simulink model "codificacion_y_modulacion_new"  (R2024b)
settings: Solver=VariableStepAuto  StartTime=0.0  StopTime=inf  RelTol=1e-3
undefined symbols (not defined in the file or in its folder): r
settings Model: SnapshotBufferSize=1000  SnapshotInterval=1000  Creator=SALA 321  LastModifiedBy=SALA 321

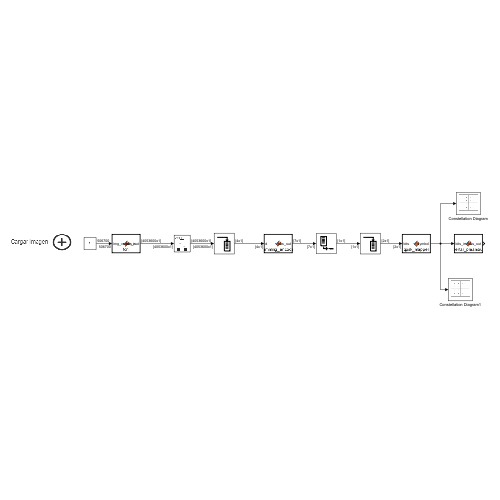
[thumbnail: Simulink's stored preview of the top-level diagram]
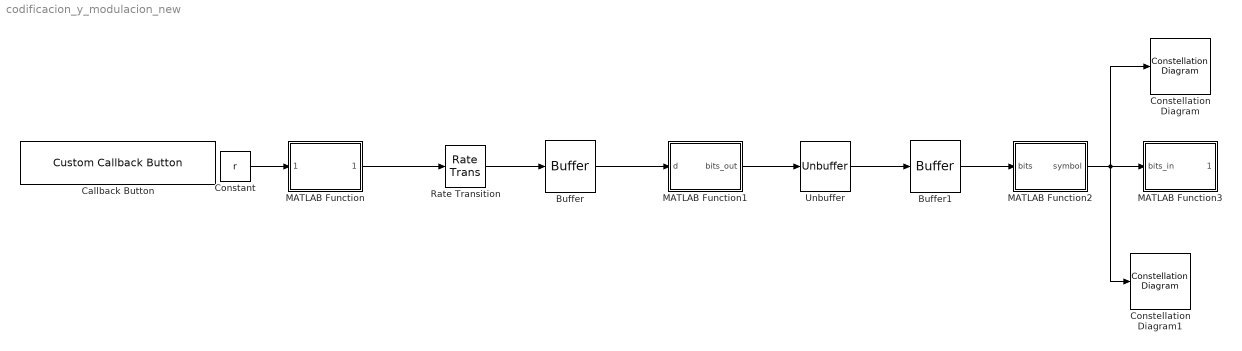
== system codificacion_y_modulacion_new ==
  Buffer : Buffer  N=4  OutputFrames=off
  Buffer1 : Buffer  N=2  OutputFrames=off
  Callback Button : CustomCallbackButton  Configuration="{\"components\":[{\"name\":\"BackgroundImageComponent\",\"settings\":{\"image\":{\"size\":[0,0],\"src\":\"default\",\"srcOrientation\":\"horizontal\"},\"position\":[0,0,1,1],\"scaleMode\":\"0\"}},{\"name\":\"ButtonStateComponent\",\"settings\":{\"buttonType\":\"momentary\",\"clickFcn\":\"[archivo, ruta] = uigetfile( ...\\n    {'*.jpg;*.jpeg;*.png;*.bmp;*.tif;*.tiff;*.gif;*.webp;*.jfif', ...\\n     'Archivos de imagen'}, ...\\n     'Seleccionar imagen');\\n\\nif isequal(archivo,0)\\n    disp('No se seleccionó imagen');\\n    return;\\nend\\n\\nrutaCompleta = fullfile(ruta, archivo);\\n\\ntry\\n    img = imread(rutaCompleta);\\ncatch\\n    errordlg('Formato no soportado por la versión de MATLAB','Error');\\n    return;\\nend\\n\\nif ndims(img) ~= 3 || size(img,3) ~= 3\\n    errordlg('La imagen debe ser RGB','Error');\\n    return;\\nend\\n\\n\\nalto = size(img,1);\\nancho = size(img,2);\\n\\nif alto < 492 || ancho < 740\\n    errordlg('La imagen debe tener mínimo 740x492 pixeles','Error');\\n    return;\\nend\\n\\nimgGray = rgb2gray(img);\\n\\nniveles = 16;              % Número de niveles de cuantización\\ndelta = 256\\/niveles;       % Paso de cuantización\\n\\nimgCuant = floor(double(img)\\/delta)*delta + delta\\/2;\\nimgCuant = uint8(imgCuant);\\n\\nassignin('base','imagen_original',img);\\nassignin('base','imagen_gris',imgGray);\\nassignin('base','imagen_cuantizada',imgCuant);\\n\\nr = reshape(imgGray,1,[]);\\nassignin('base','r',r);\\n\\ndisp(['Imagen cargada correctamente: ', archivo]);\\ndisp(['Tamaño: ', num2str(ancho), 'x', num2str(alto)]);\\ndisp(['Vector serializado r → tamaño: ', mat2str(size(r))]);\\n\\nfigure(2)\\nsubplot(1,2,1)\\nimshow(img)\\ntitle('Imagen Original')\\n\\nsubplot(1,2,2)\\nimshow(imgCuant)\\ntitle('Imagen Comprimida')\",\"image\":{\"size\":[180,45],\"srcOrientation\":\"Right\"},\"onValue\":1,\"position\":[0,0,1,1],\"pressDelay\":\"500\",\"pressFcn\":\"\",\"repeatInterval\":\"0\",\"states\":[{\"horizontalAlignment\":\"left\",\"image\":{\"position\":[0,0.62,0.25,1],\"size\":[0.25,1],\"src\":\"data:image\\/png;base64,iVBORw0KGgoAAAANSUhEUgAAAgAAAAIACAMAAADDpiTIAAAAA3NCSVQICAjb4U\\/gAAAACXBIWXMAAA3XAAAN1wFCKJt4AAAAGXRFWHRTb2Z0d2FyZQB3d3cuaW5rc2NhcGUub3Jnm+48GgAAAm1QTFRF\\/\\/\\/\\/AAAAAAAAAAAAAAAAAAAAAAAAAAAAAAAAAAAAAAAAAAAAAAAAAAAAAAAAAAAAAAAAAAAAAAAAAAAAAAAAAAAAAAAAAAAAAAAAAAAAAAAAAAAAAAAAAAAAAAAAAAAAAAAAAAAAAAAAAAAAAAAAAAAAAAAAAAAAAAAAAAAAAAAAAAAAAAAAAAAAAAAAAAAAAAAAAAAAAAAAAAAAAAAAAAAAAAAAAAAAAAAAAAAAAAAAAA ...(+11910 chars)\",\"srcOrientation\":\"Right\"},\"label\":{\"color\":[0,0,0],\"icon\":{\"size\":[0,0],\"src\":[],\"srcOrientation\":\"Right\"},\"iconOffset\":0,\"iconPlacement\":\"left\",\"opacity\":1,\"show\":true,\"text\":{\"content\":\"Cargar Imagen\",\"font\":\"Helvetica\"}},\"labelOffset\":[-0.02,0.09],\"verticalAlignment\":\"middle\"},{\"horizontalAlignment\":\"center\",\"image\":{\"position\":[0.05,0.015,0.98,0.9],\"size\":[0.98,0.9],\"src\":\"data:image\\/svg+xml;base64,PHN2ZyB4bWxucz0iaHR0cDovL3d3dy53My5vcmcvMjAwMC9zdmciIHhtbG5zOnhsaW5rPSJodHRwOi8vd3d3LnczLm9yZy8xOTk5L3hsaW5rIiB2aWV3Qm94PSIwIDAgMTc3LjI1IDQwLjg4Ij48ZGVmcz48c3R5bGU+LmNscy0xe2ZpbGw6dXJsKCNyYWRpYWwtZ3JhZGllbnQpO30uY2xzLTJ7ZmlsbDp1cmwoI2xpbmVhci1ncmFkaWVudCk7fS5jbHMtM3tmaWxsOnVybCgjbGluZWFyLWdyYWRpZW50LTIpO308L3N0eWxlPjxyYWRpYWxHcmFkaWVudCBpZD0icmFkaWFsLWdyYWRpZW50IiBjeD0iOTAuMDkiIGN5PSIyMi42NiIgcj0i ...(+2216 chars)\",\"srcOrientation\":\"Right\"},\"label\":{\"color\":[1,1,1],\"icon\":{\"size\":[0,0],\"src\":[],\"srcOrientation\":\"Right\"},\"iconOffset\":0,\"iconPlacement\":\"left\",\"opacity\":1,\"show\":true,\"text\":{\"content\":\"Callback Button\",\"font\":\"Helvetica\"}},\"labelOffset\":[0,0],\"verticalAlignment\":\"middle\"},{\"horizontalAlignment\":\"center\",\"image\":{\"position\":[0.05,0.015,0.98,0.9],\"size\":[0.98,0.9],\"src\":\"data:image\\/svg+xml;base64,PHN2ZyB4bWxucz0iaHR0cDovL3d3dy53My5vcmcvMjAwMC9zdmciIHhtbG5zOnhsaW5rPSJodHRwOi8vd3d3LnczLm9yZy8xOTk5L3hsaW5rIiB2aWV3Qm94PSIwIDAgMTc3LjI1IDQwLjg4Ij48ZGVmcz48c3R5bGU+LmNscy0xe2ZpbGw6dXJsKCNyYWRpYWwtZ3JhZGllbnQpO30uY2xzLTJ7ZmlsbDp1cmwoI2xpbmVhci1ncmFkaWVudCk7fS5jbHMtM3tmaWxsOnVybCgjbGluZWFyLWdyYWRpZW50LTIpO308L3N0eWxlPjxyYWRpYWxHcmFkaWVudCBpZD0icmFkaWFsLWdyYWRpZW50IiBjeD0iOTAuMDkiIGN5PSIyMi42NiIgcj0i ...(+2212 chars)\",\"srcOrientation\":\"Right\"},\"label\":{\"color\":[1,1,0.78,1],\"icon\":{\"size\":[0,0],\"src\":[],\"srcOrientation\":\"Right\"},\"iconOffset\":0,\"iconPlacement\":\"left\",\"opacity\":1,\"show\":true,\"text\":{\"content\":\"Callback Button\",\"font\":\"Helvetica\"}},\"labelOffset\":[-0.025,0],\"verticalAlignment\":\"middle\"},{\"horizontalAlignment\":\"center\",\"image\":{\"position\":[0.05,0.015,0.98,0.9],\"size\":[0.98,0.9],\"src\":\"data:image\\/svg+xml;base64,PHN2ZyB4bWxucz0iaHR0cDovL3d3dy53My5vcmcvMjAwMC9zdmciIHhtbG5zOnhsaW5rPSJodHRwOi8vd3d3LnczLm9yZy8xOTk5L3hsaW5rIiB2aWV3Qm94PSIwIDAgMTc3LjI1IDQwLjg4Ij48ZGVmcz48c3R5bGU+LmNscy0xe2ZpbGw6dXJsKCNyYWRpYWwtZ3JhZGllbnQpO30uY2xzLTJ7ZmlsbDp1cmwoI2xpbmVhci1ncmFkaWVudCk7fS5jbHMtM3tmaWxsOnVybCgjbGluZWFyLWdyYWRpZW50LTIpO308L3N0eWxlPjxyYWRpYWxHcmFkaWVudCBpZD0icmFkaWFsLWdyYWRpZW50IiBjeD0iOTAuMDkiIGN5PSIyMi42NiIgcj0i ...(+2216 chars)\",\"srcOrientation\":\"Right\"},\"label\":{\"color\":[1,1,0.78,1],\"icon\":{\"size\":[0,0],\"src\":[],\"srcOrientation\":\"Right\"},\"iconOffset\":0,\"iconPlacement\":\"left\",\"opacity\":1,\"show\":true,\"text\":{\"content\":\"Callback Button\",\"font\":\"Helvetica\"}},\"labelOffset\":[0,0],\"verticalAlignment\":\"middle\"}]}},{\"name\":\"ForegroundImageComponent\",\"settings\":{\"image\":{\"size\":[0,0],\"src\":\"default\",\"srcOrientation\":\"horizontal\"},\"isForeground\":1,\"position\":[0,0,1,1],\"scaleMode\":\"0\"}}],\"settings\":{\"BindingType\":\"param\",\"aspectRatio\":3.7777777777777777,\"backgroundColor\":[255,255,255,\"1\"],\"backgroundOffset\":0,\"backgroundOpacity\":1,\"fixedAspectRatio\":\"on\",\"foregroundColor\":[252,252,196],\"showBackgroundColor\":false,\"variant\":\"callback\",\"version\":\"R2024b\"},\"type\":\"Button\"}"
  Constant : Constant  Value=r
  Constellation Diagram : ConstellationDiagram  WindowPosition=[348.000000,86.000000,600.000000,560.000000,]  Visible=on  ScopeFrameLocation=window  SymbolsToDisplaySource=Property  SymbolsToDisplay=1000  ReferenceConstellation=QPSK  XLimits=[-2.14,2.15]  YLimits=[-1.38,1.38]  ShowReferenceConstellation=off
  Constellation Diagram1 : ConstellationDiagram  WindowPosition=[382.000000,84.000000,600.000000,600.000000,]  Visible=on  ScopeFrameLocation=window  ReferenceConstellation=QPSK  ShowReferenceConstellation=off
  MATLAB Function : MATLAB Function  TreatAsAtomicUnit=on
  MATLAB Function1 : MATLAB Function  TreatAsAtomicUnit=on
  MATLAB Function2 : MATLAB Function  TreatAsAtomicUnit=on
  MATLAB Function3 : MATLAB Function  TreatAsAtomicUnit=on
  Rate Transition : RateTransition  OutPortSampleTime=1000000000000000000000000000000
  Unbuffer : Unbuffer
  wires:
  MATLAB Function/1(bits_out) -> Rate Transition/1
  Rate Transition/1 -> Buffer/1
  Constant/1 -> MATLAB Function/1(img_vector_in)
  Buffer/1 -> MATLAB Function1/1(d)
  Buffer1/1 -> MATLAB Function2/1(bits)
  Unbuffer/1 -> Buffer1/1
  MATLAB Function1/1(bits_out) -> Unbuffer/1
  MATLAB Function2/1(symbol) -> MATLAB Function3/1(bits_in), Constellation Diagram/1, Constellation Diagram1/1

== matlab function codificacion_y_modulacion_new/MATLAB Function ==
  data: bits_out output; img_vector_in input
function bits_out = fcn(img_vector_in)
% #codegen
% img_vector_in: Se espera un vector fila con los valores de los píxeles

%% 1. Asegurar que sea uint8
% Si el vector viene de otro bloque, lo forzamos a entero de 8 bits
img_uint8 = uint8(img_vector_in);

%% 2. Convertir cada píxel a 8 bits
% Si recibes un vector de 10,000 píxeles, la salida será de 80,000 bits.
num_pixels = numel(img_uint8);

% Importante: Si la entrada es un vector fila, lo ponemos en columna para procesar
pixel_col = img_uint8(:);

% Matriz para guardar los bits (8 bits por cada píxel)
bits_matrix = zeros(num_pixels, 8, 'uint8');

for b = 1:8
    % Extraemos los bits del MSB (bit 8) al LSB (bit 1)
    bits_matrix(:, 9-b) = bitget(pixel_col, b); 
end

%% 3. Aplanamiento para salida serial
% Transponemos para que los bits de un mismo píxel queden seguidos
temp = bits_matrix';
all_bits = temp(:);

% Salida como vector columna de bits (compatible con Unbuffer)
bits_out = single(all_bits);

end

== matlab function codificacion_y_modulacion_new/MATLAB Function2 ==
  data: bits input; symbol output
function symbol = qpsk_mapper(bits)
%#codegen
% bits: vector de 2x1 que contiene [b1; b2]
% symbol: símbolo complejo QPSK

b1 = bits(1);
b2 = bits(2);

if b1==0 && b2==0
    symbol = (1 + 1j)/sqrt(2);

elseif b1==0 && b2==1
    symbol = (-1 + 1j)/sqrt(2);

elseif b1==1 && b2==1
    symbol = (-1 - 1j)/sqrt(2);

else % 10
    symbol = (1 - 1j)/sqrt(2);

end

end

== matlab function codificacion_y_modulacion_new/MATLAB Function3 ==
  data: bits_in input; bits_out output
function bits_out = insertar_preambulo(bits_in)
%#codegen

% Preámbulo conocido (32 bits)
preamble = [1 0 1 0 1 0 1 0 ...
            1 1 0 0 1 1 0 0 ...
            1 0 1 0 1 0 1 0 ...
            1 1 0 0 1 1 0 0];

% Asegurar que bits_in sea vector fila
bits_in = bits_in(:)';

% Concatenar preámbulo + datos
bits_out = [preamble bits_in];

end

== matlab function codificacion_y_modulacion_new/MATLAB Function1 ==
  data: d input; bits_out output
function bits_out = hamming_encoder(d)
%#codegen

% Asegurar vector columna
d = d(:);

% Preasignar salida (7 bits)
bits_out = zeros(7,1);

d1 = d(1);
d2 = d(2);
d3 = d(3);
d4 = d(4);

% Bits de paridad
p1 = xor(xor(d1,d2),d4);
p2 = xor(xor(d1,d3),d4);
p3 = xor(xor(d2,d3),d4);

% Palabra codificada Hamming (7,4)
bits_out(1) = p1;
bits_out(2) = p2;
bits_out(3) = d1;
bits_out(4) = p3;
bits_out(5) = d2;
bits_out(6) = d3;
bits_out(7) = d4;

end
